simulink model "pmsg_wind_turbine_simpCURRENT"  (R2022a)
settings: Solver=ode23tb  StartTime=0.0  StopTime=3.5  FixedStep=1e-4  MaxStep=1e-6  RelTol=1e-3
undefined symbols (not defined in the file): Ci, current, Lb, y
libraries: spsCurrentMeasurementLib x2, spsSeriesRLCBranchLib x2, spsVoltageMeasurementLib x2, spsControlledCurrentSourceLib x1, simulink x1, spsDCVoltageSourceLib x1, spsDiodeLib x1, spsMosfetLib x1, slpidlib x1, spsPWMGeneratorDCDCLib x1, eePowerMeasurement x1, spspowerguiLib x1
settings Model: Creator=Taysa Banik  LastModifiedBy=LICON
settings SolverCC: ZeroCrossAlgorithm=Adaptive
settings DebuggingCC: MaxConsecutiveZCsMsg=warning  MaskedZcDiagnostic=none  IgnoredZcDiagnostic=none  MultiTaskCondExecSysMsg=warning  MultiTaskRateTransMsg=warning  ModelReferenceExtraNoncontSigs=warning

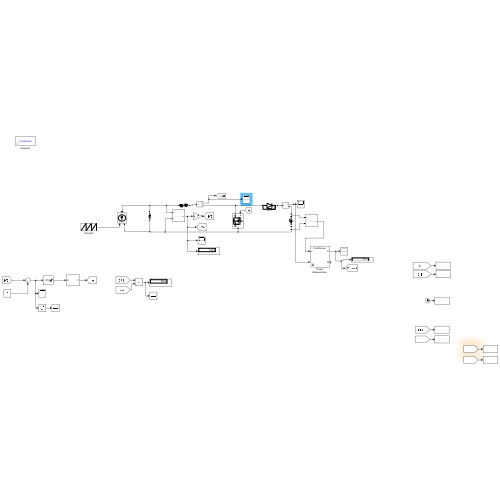
[thumbnail: Simulink's stored preview of the top-level diagram]
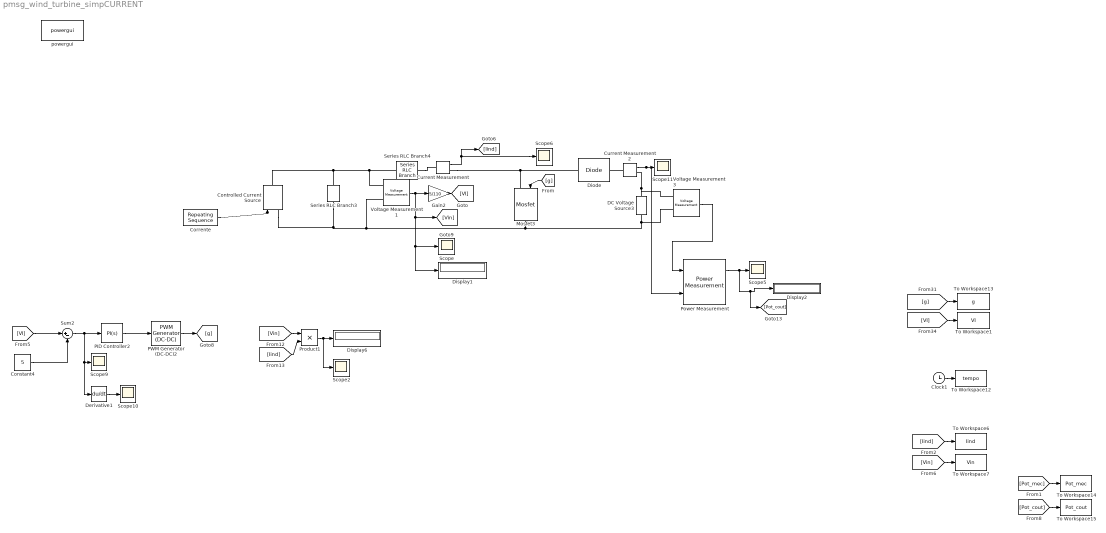
== system pmsg_wind_turbine_simpCURRENT ==
  Clock1 : Clock
  Constant4 : Constant  Value=5
  Controlled Current Source : spsControlledCurrentSourceLib/Controlled Current Source  Initialize=on  Source_Type=AC  Amplitude=0  Phase=0  Frequency=0  Measurements=None
  Corrente : simulink/Sources/Repeating Sequence  rep_seq_t=[y]  rep_seq_y=[current]
  Current Measurement : spsCurrentMeasurementLib/Current Measurement  PhasorSimulation=off  OutputType=Complex  PSBequivalent=0
  Current Measurement2 : spsCurrentMeasurementLib/Current Measurement  PhasorSimulation=off  OutputType=Complex  PSBequivalent=0
  DC Voltage Source3 : spsDCVoltageSourceLib/DC Voltage Source  Amplitude=400  Measurements=Voltage
  Derivative1 : Derivative
  Diode : spsDiodeLib/Diode  Ron=0.001  Lon=0  Vf=0.1  IC=0  UseSnubber=0  Rs=50000  Cs=inf  Measurements=off
  Display1 : Display
  Display2 : Display
  Display6 : Display
  Gain2 : Gain  Gain=5/110
  Mosfet3 : spsMosfetLib/Mosfet  Ron=0.001  Lon=0  Rd=0.01  Vfd=0  IC=0  Rs=1e5  Cs=inf  Measurements=off
  PID Controller2 : slpidlib/PID Controller  Controller=PI  Form=Parallel  TimeDomain=Continuous-time  UseExternalTs=off  SampleTime=-1  IntegratorMethod=Forward Euler  FilterMethod=Forward Euler  ControllerParametersSource=internal  P=0.1928  I=11.6277  UseKiTs=off  D=0  N=100  UseFilter=on  TunerSelectOption=Frequency Response Based  InitialConditionSource=internal  InitialConditionForIntegrator=0  InitialConditionForFilter=0  DifferentiatorICPrevScaledInput=0  ExternalReset=none  TrackingMode=off  Kt=1  LimitOutput=on  SatLimitsSource=internal  UpperSaturationLimit=0.95  LowerSaturationLimit=0  LinearizeAsGain=on  AntiWindupMode=none  Kb=1  POutMin=[]  POutMax=[]  IOutMin=[]  IOutMax=[]  DOutMin=[]  DOutMax=[]  NOutMin=[]  NOutMax=[]  SumOutMin=[]  SumOutMax=[]  SaturationOutMin=[]  SaturationOutMax=[]  PParamMin=[]  PParamMax=[]  IParamMin=[]  IParamMax=[]  DParamMin=[]  DParamMax=[]  NParamMin=[]  NParamMax=[]  KbParamMin=[]  KbParamMax=[]  KtParamMin=[]  KtParamMax=[]  KbOutMin=[]  KbOutMax=[]  KtOutMin=[]  KtOutMax=[]  IntegratorOutMin=[]  IntegratorOutMax=[]  FilterOutMin=[]  FilterOutMax=[]  SumI1OutMin=[]  SumI1OutMax=[]  SumI2OutMin=[]  SumI2OutMax=[]  SumI3OutMin=[]  SumI3OutMax=[]  SumI4OutMin=[]  SumI4OutMax=[]  SumDOutMin=[]  SumDOutMax=[]  DifferentiatorOutMin=[]  DifferentiatorOutMax=[]  FilterDiffOutCoefMin=[]  FilterDiffOutCoefMax=[]  ReciprocalOutMin=[]  ReciprocalOutMax=[]  SumDenOutMin=[]  SumDenOutMax=[]  SumNumOutMin=[]  SumNumOutMax=[]  DivideOutMin=[]  DivideOutMax=[]  UdiffTsProdOutMin=[]  UdiffTsProdOutMax=[]  NTsProdOutMin=[]  NTsProdOutMax=[]  UintegralTsProdOutMin=[]  UintegralTsProdOutMax=[]  UngainTsProdOutMin=[]  UngainTsProdOutMax=[]  IntegratorContinuousStateAttributes=''  IntegratorStateMustResolveToSignalObject=off  IntegratorRTWStateStorageClass=Auto  FilterContinuousStateAttributes=''  FilterStateMustResolveToSignalObject=off  FilterRTWStateStorageClass=Auto  ParallelPVariant=InternalParameters  IdealPVariant=Disabled  IVariant=InternalParameters  DVariant=Disabled  IntegratorVariant=Continuous  SatVariant=Enabled  AWVariant=Passthrough  PCopyVariant=Disabled  TRVariant=Disabled  FdbkBlocksVariant=Forward  IdealPFdbkVariant=Disabled  SatFdbkVariant=Disabled  DerivativeFilterVariant=Disabled  NVariant=Disabled  NCopyVariant=Disabled_SignalSpec  FilterICVariant=Disabled  IntegratorICVariant=InternalICs  ExternalResetVariant=Disabled  TRSumVariant=Passthrough  SumFdbkVariant=Disabled  SumVariant=Sum_PI  TsampFilterVariant=InternalTs  TsampNgainVariant=Passthrough  TsampIntegralVariant=Passthrough  ExternalSaturationOutDataTypeStr=Inherit: Same as second input  aMode=0
  PWM Generator (DC-DC)2 : spsPWMGeneratorDCDCLib/PWM Generator (DC-DC)  Fsw=30000  Ts=1e-6
  Power Measurement : eePowerMeasurement/Power Measurement  LabelModeActiveChoice=Continuous  F=79.33  K=[0]  Ts=0
      settings: SourceProductBaseCode=PS
  Product1 : Product
  Scope{,2,5..6,9..11} (7 alike) : Scope
  Series RLC Branch3 : spsSeriesRLCBranchLib/Series RLC Branch  LConnTagsString=__new0  RConnTagsString=__new0  BranchType=C  Resistance=1  Inductance=1e-3  SetiL0=off  InitialCurrent=0  Capacitance=Ci  Setx0=on  InitialVoltage=100  Measurements=None
  Series RLC Branch4 : spsSeriesRLCBranchLib/Series RLC Branch  LConnTagsString=__new0  RConnTagsString=__new0  BranchType=RL  Resistance=1  Inductance=Lb  SetiL0=off  InitialCurrent=0  Capacitance=1e-3  Setx0=off  InitialVoltage=0  Measurements=None
  Sum2 : Sum  Inputs=|+-
  To Workspace1 : ToWorkspace  VariableName=VI  SampleTime=1e-6
  To Workspace12 : ToWorkspace  VariableName=tempo  SampleTime=1e-6
  To Workspace13 : ToWorkspace  VariableName=g  SampleTime=1e-6
  To Workspace14 : ToWorkspace  VariableName=Pot_mec  SampleTime=1e-6
  To Workspace15 : ToWorkspace  VariableName=Pot_cout  SampleTime=1e-6
  To Workspace6 : ToWorkspace  VariableName=Iind  SampleTime=1e-6
  To Workspace7 : ToWorkspace  VariableName=Vin  SampleTime=1e-6
  Voltage Measurement1 : spsVoltageMeasurementLib/Voltage Measurement  PhasorSimulation=off  OutputType=Complex  PSBequivalent=0
  Voltage Measurement3 : spsVoltageMeasurementLib/Voltage Measurement  PhasorSimulation=off  OutputType=Complex  PSBequivalent=0
  powergui : spspowerguiLib/powergui  Priority=1  SimulationMode=Continuous  SampleTime=50e-6  frequency=60  Iterations=50  frequencyindice=0  Pbase=100e6  ErrMax=1e-4  UnitsV=kV  UnitsW=MW  buscounter=0  FunctionMessages=off  echomessages=off  EnableUseOfTLC=off  CurrentSourceSwitches=off  DisableSnubberDevices=off  DisableRonSwitches=off  DisableVfSwitches=off  DisplayEquations=off  AutomaticDiscreteSolvers=off  SolverType=Tustin/Backward Euler (TBE)  Interpol=off  ExternalGateDelay=off  methode=off  Ts=100  x0status=blocks  SPID=on  SwTol=0  HookPort=off  NonlinearTolerance=1e-4  nMaxIteration=100  ContinueOnMaxIteration=off  RestoreLinks=warning  ResistiveCurrentMeasurement=off  Frange=[0:2:500]  Ylog=off  Xlog=on  ShowGrid=off  save=off  variable=ZData  structure=0  ZoomFFT=off  StartTime=0.0  cycles=1  DisplayStyle=1  fundamental=60  FreqAxis=off  MaxFrequency=1000  frequencyindicesteady=1  RmsSteady=1  display=off
  wires:
  Voltage Measurement1/1 -> Gain2/1, [Vin], Scope/1, Display1/1
  [g] -> Mosfet3/1
  Gain2/1 -> [VI]
  [VI] -> To Workspace1/1
  [g] -> To Workspace13/1
  Clock1/1 -> To Workspace12/1
  Current Measurement/1 -> [Iind], Scope6/1
  [Iind] -> To Workspace6/1
  Constant4/1 -> Sum2/2
  [VI] -> Sum2/1
  PID Controller2/1 -> PWM Generator (DC-DC)2/1
  Derivative1/1 -> Scope10/1
  PWM Generator (DC-DC)2/1 -> [g]
  Sum2/1 -> Derivative1/1, Scope9/1, PID Controller2/1
  [Vin] -> To Workspace7/1
  [Pot_mec] -> To Workspace14/1
  Current Measurement2/1 -> Power Measurement/2, Scope11/1
  Voltage Measurement3/1 -> Power Measurement/1
  Power Measurement/1 -> [Pot_cout], Display2/1, Scope5/1
  [Pot_cout] -> To Workspace15/1
  [Vin] -> Product1/1
  [Iind] -> Product1/2
  Product1/1 -> Scope2/1, Display6/1
  Corrente/1 -> Controlled Current Source/1
  connections:
  Mosfet3/LConn1 -- Current Measurement/RConn1 -- Diode/LConn1
  Voltage Measurement1/LConn1 -- Series RLC Branch4/LConn1 -- Controlled Current Source/RConn1 -- Series RLC Branch3/LConn1
  Series RLC Branch4/RConn1 -- Current Measurement/LConn1
  Current Measurement2/LConn1 -- Diode/RConn1
  DC Voltage Source3/RConn1 -- Current Measurement2/RConn1 -- Voltage Measurement3/LConn1
  Voltage Measurement3/LConn2 -- Controlled Current Source/LConn1 -- Series RLC Branch3/RConn1 -- Voltage Measurement1/LConn2 -- Mosfet3/RConn1 -- DC Voltage Source3/LConn1
